simulink library "UndergraduateResearch"  (Simulink 8.1)
settings: Solver=ode45  StartTime=0.0  StopTime=10.0  RelTol=1e-3
undefined symbols (not defined in the file or in its folder): datafiI, datafiQ, i, magnitude
libraries: commchan3 x40, UndergraduateResearch x35, dspxfrm3 x6, dspstat3 x4, dspmtrx3 x4, commseqgen2 x4, dspindex x2, simulink x2, dspbuff3 x1
(part 2 of 2)

== system UndergraduateResearch/Frame Based Signal Generator (Any Sampling Frequency)/Noise Addition/AWGN channel16 ==
  Signal : Inport
  AWGN Channel : commchan3/AWGN Channel  InputProcessing=Columns as channels (frame based)  seed=16  noiseMode="Signal to noise ratio  (SNR)"  EbNodB=10  EsNodB=10  SNRdB=-20  bitsPerSym=1  Ps=1  Tsym=1  variance=1
  Frame Conversion : FrameConversion  OutFrame=Sample-based
  SIgnal+Noise : Outport
  wires:
  Signal/1 -> AWGN Channel/1
  AWGN Channel/1 -> Frame Conversion/1
  Frame Conversion/1 -> SIgnal+Noise/1

== system UndergraduateResearch/Frame Based Signal Generator (Any Sampling Frequency)/Noise Addition/AWGN channel17 ==
  Signal : Inport
  AWGN Channel : commchan3/AWGN Channel  InputProcessing=Columns as channels (frame based)  seed=17  noiseMode="Signal to noise ratio  (SNR)"  EbNodB=10  EsNodB=10  SNRdB=-20  bitsPerSym=1  Ps=1  Tsym=1  variance=1
  Frame Conversion : FrameConversion  OutFrame=Sample-based
  SIgnal+Noise : Outport
  wires:
  Signal/1 -> AWGN Channel/1
  AWGN Channel/1 -> Frame Conversion/1
  Frame Conversion/1 -> SIgnal+Noise/1

== system UndergraduateResearch/Frame Based Signal Generator (Any Sampling Frequency)/Noise Addition/AWGN channel18 ==
  Signal : Inport
  AWGN Channel : commchan3/AWGN Channel  InputProcessing=Columns as channels (frame based)  seed=18  noiseMode="Signal to noise ratio  (SNR)"  EbNodB=10  EsNodB=10  SNRdB=-20  bitsPerSym=1  Ps=1  Tsym=1  variance=1
  Frame Conversion : FrameConversion  OutFrame=Sample-based
  SIgnal+Noise : Outport
  wires:
  Signal/1 -> AWGN Channel/1
  AWGN Channel/1 -> Frame Conversion/1
  Frame Conversion/1 -> SIgnal+Noise/1

== system UndergraduateResearch/Frame Based Signal Generator (Any Sampling Frequency)/Noise Addition/AWGN channel19 ==
  Signal : Inport
  AWGN Channel : commchan3/AWGN Channel  InputProcessing=Columns as channels (frame based)  seed=19  noiseMode="Signal to noise ratio  (SNR)"  EbNodB=10  EsNodB=10  SNRdB=-20  bitsPerSym=1  Ps=1  Tsym=1  variance=1
  Frame Conversion : FrameConversion  OutFrame=Sample-based
  SIgnal+Noise : Outport
  wires:
  Signal/1 -> AWGN Channel/1
  AWGN Channel/1 -> Frame Conversion/1
  Frame Conversion/1 -> SIgnal+Noise/1

== system UndergraduateResearch/Frame Based Signal Generator (Any Sampling Frequency)/Noise Addition/AWGN channel2 ==
  Signal : Inport
  AWGN Channel : commchan3/AWGN Channel  InputProcessing=Columns as channels (frame based)  seed=2  noiseMode="Signal to noise ratio  (SNR)"  EbNodB=10  EsNodB=10  SNRdB=-20  bitsPerSym=1  Ps=1  Tsym=1  variance=1
  Frame Conversion : FrameConversion  OutFrame=Sample-based
  SIgnal+Noise : Outport
  wires:
  Signal/1 -> AWGN Channel/1
  AWGN Channel/1 -> Frame Conversion/1
  Frame Conversion/1 -> SIgnal+Noise/1

== system UndergraduateResearch/Frame Based Signal Generator (Any Sampling Frequency)/Noise Addition/AWGN channel20 ==
  Signal : Inport
  AWGN Channel : commchan3/AWGN Channel  InputProcessing=Columns as channels (frame based)  seed=20  noiseMode="Signal to noise ratio  (SNR)"  EbNodB=10  EsNodB=10  SNRdB=-20  bitsPerSym=1  Ps=1  Tsym=1  variance=1
  Frame Conversion : FrameConversion  OutFrame=Sample-based
  SIgnal+Noise : Outport
  wires:
  Signal/1 -> AWGN Channel/1
  AWGN Channel/1 -> Frame Conversion/1
  Frame Conversion/1 -> SIgnal+Noise/1

== system UndergraduateResearch/Frame Based Signal Generator (Any Sampling Frequency)/Noise Addition/AWGN channel21 ==
  Signal : Inport
  AWGN Channel : commchan3/AWGN Channel  InputProcessing=Columns as channels (frame based)  seed=21  noiseMode="Signal to noise ratio  (SNR)"  EbNodB=10  EsNodB=10  SNRdB=-20  bitsPerSym=1  Ps=1  Tsym=1  variance=1
  Frame Conversion : FrameConversion  OutFrame=Sample-based
  SIgnal+Noise : Outport
  wires:
  Signal/1 -> AWGN Channel/1
  AWGN Channel/1 -> Frame Conversion/1
  Frame Conversion/1 -> SIgnal+Noise/1

== system UndergraduateResearch/Frame Based Signal Generator (Any Sampling Frequency)/Noise Addition/AWGN channel22 ==
  Signal : Inport
  AWGN Channel : commchan3/AWGN Channel  InputProcessing=Columns as channels (frame based)  seed=22  noiseMode="Signal to noise ratio  (SNR)"  EbNodB=10  EsNodB=10  SNRdB=-20  bitsPerSym=1  Ps=1  Tsym=1  variance=1
  Frame Conversion : FrameConversion  OutFrame=Sample-based
  SIgnal+Noise : Outport
  wires:
  Signal/1 -> AWGN Channel/1
  AWGN Channel/1 -> Frame Conversion/1
  Frame Conversion/1 -> SIgnal+Noise/1

== system UndergraduateResearch/Frame Based Signal Generator (Any Sampling Frequency)/Noise Addition/AWGN channel23 ==
  Signal : Inport
  AWGN Channel : commchan3/AWGN Channel  InputProcessing=Columns as channels (frame based)  seed=23  noiseMode="Signal to noise ratio  (SNR)"  EbNodB=10  EsNodB=10  SNRdB=-20  bitsPerSym=1  Ps=1  Tsym=1  variance=1
  Frame Conversion : FrameConversion  OutFrame=Sample-based
  SIgnal+Noise : Outport
  wires:
  Signal/1 -> AWGN Channel/1
  AWGN Channel/1 -> Frame Conversion/1
  Frame Conversion/1 -> SIgnal+Noise/1

== system UndergraduateResearch/Frame Based Signal Generator (Any Sampling Frequency)/Noise Addition/AWGN channel24 ==
  Signal : Inport
  AWGN Channel : commchan3/AWGN Channel  InputProcessing=Columns as channels (frame based)  seed=24  noiseMode="Signal to noise ratio  (SNR)"  EbNodB=10  EsNodB=10  SNRdB=-20  bitsPerSym=1  Ps=1  Tsym=1  variance=1
  Frame Conversion : FrameConversion  OutFrame=Sample-based
  SIgnal+Noise : Outport
  wires:
  Signal/1 -> AWGN Channel/1
  AWGN Channel/1 -> Frame Conversion/1
  Frame Conversion/1 -> SIgnal+Noise/1

== system UndergraduateResearch/Frame Based Signal Generator (Any Sampling Frequency)/Noise Addition/AWGN channel25 ==
  Signal : Inport
  AWGN Channel : commchan3/AWGN Channel  InputProcessing=Columns as channels (frame based)  seed=25  noiseMode="Signal to noise ratio  (SNR)"  EbNodB=10  EsNodB=10  SNRdB=-20  bitsPerSym=1  Ps=1  Tsym=1  variance=1
  Frame Conversion : FrameConversion  OutFrame=Sample-based
  SIgnal+Noise : Outport
  wires:
  Signal/1 -> AWGN Channel/1
  AWGN Channel/1 -> Frame Conversion/1
  Frame Conversion/1 -> SIgnal+Noise/1

== system UndergraduateResearch/Frame Based Signal Generator (Any Sampling Frequency)/Noise Addition/AWGN channel26 ==
  Signal : Inport
  AWGN Channel : commchan3/AWGN Channel  InputProcessing=Columns as channels (frame based)  seed=26  noiseMode="Signal to noise ratio  (SNR)"  EbNodB=10  EsNodB=10  SNRdB=-20  bitsPerSym=1  Ps=1  Tsym=1  variance=1
  Frame Conversion : FrameConversion  OutFrame=Sample-based
  SIgnal+Noise : Outport
  wires:
  Signal/1 -> AWGN Channel/1
  AWGN Channel/1 -> Frame Conversion/1
  Frame Conversion/1 -> SIgnal+Noise/1

== system UndergraduateResearch/Frame Based Signal Generator (Any Sampling Frequency)/Noise Addition/AWGN channel27 ==
  Signal : Inport
  AWGN Channel : commchan3/AWGN Channel  InputProcessing=Columns as channels (frame based)  seed=27  noiseMode="Signal to noise ratio  (SNR)"  EbNodB=10  EsNodB=10  SNRdB=-20  bitsPerSym=1  Ps=1  Tsym=1  variance=1
  Frame Conversion : FrameConversion  OutFrame=Sample-based
  SIgnal+Noise : Outport
  wires:
  Signal/1 -> AWGN Channel/1
  AWGN Channel/1 -> Frame Conversion/1
  Frame Conversion/1 -> SIgnal+Noise/1

== system UndergraduateResearch/Frame Based Signal Generator (Any Sampling Frequency)/Noise Addition/AWGN channel28 ==
  Signal : Inport
  AWGN Channel : commchan3/AWGN Channel  InputProcessing=Columns as channels (frame based)  seed=28  noiseMode="Signal to noise ratio  (SNR)"  EbNodB=10  EsNodB=10  SNRdB=-20  bitsPerSym=1  Ps=1  Tsym=1  variance=1
  Frame Conversion : FrameConversion  OutFrame=Sample-based
  SIgnal+Noise : Outport
  wires:
  Signal/1 -> AWGN Channel/1
  AWGN Channel/1 -> Frame Conversion/1
  Frame Conversion/1 -> SIgnal+Noise/1

== system UndergraduateResearch/Frame Based Signal Generator (Any Sampling Frequency)/Noise Addition/AWGN channel29 ==
  Signal : Inport
  AWGN Channel : commchan3/AWGN Channel  InputProcessing=Columns as channels (frame based)  seed=29  noiseMode="Signal to noise ratio  (SNR)"  EbNodB=10  EsNodB=10  SNRdB=-20  bitsPerSym=1  Ps=1  Tsym=1  variance=1
  Frame Conversion : FrameConversion  OutFrame=Sample-based
  SIgnal+Noise : Outport
  wires:
  Signal/1 -> AWGN Channel/1
  AWGN Channel/1 -> Frame Conversion/1
  Frame Conversion/1 -> SIgnal+Noise/1

== system UndergraduateResearch/Frame Based Signal Generator (Any Sampling Frequency)/Noise Addition/AWGN channel3 ==
  Signal : Inport
  AWGN Channel : commchan3/AWGN Channel  InputProcessing=Columns as channels (frame based)  seed=3  noiseMode="Signal to noise ratio  (SNR)"  EbNodB=10  EsNodB=10  SNRdB=-20  bitsPerSym=1  Ps=1  Tsym=1  variance=1
  Frame Conversion : FrameConversion  OutFrame=Sample-based
  SIgnal+Noise : Outport
  wires:
  Signal/1 -> AWGN Channel/1
  AWGN Channel/1 -> Frame Conversion/1
  Frame Conversion/1 -> SIgnal+Noise/1

== system UndergraduateResearch/Frame Based Signal Generator (Any Sampling Frequency)/Noise Addition/AWGN channel30 ==
  Signal : Inport
  AWGN Channel : commchan3/AWGN Channel  InputProcessing=Columns as channels (frame based)  seed=10  noiseMode="Signal to noise ratio  (SNR)"  EbNodB=10  EsNodB=10  SNRdB=-20  bitsPerSym=1  Ps=1  Tsym=1  variance=1
  Frame Conversion : FrameConversion  OutFrame=Sample-based
  SIgnal+Noise : Outport
  wires:
  Signal/1 -> AWGN Channel/1
  AWGN Channel/1 -> Frame Conversion/1
  Frame Conversion/1 -> SIgnal+Noise/1

== system UndergraduateResearch/Frame Based Signal Generator (Any Sampling Frequency)/Noise Addition/AWGN channel31 ==
  Signal : Inport
  AWGN Channel : commchan3/AWGN Channel  InputProcessing=Columns as channels (frame based)  seed=10  noiseMode="Signal to noise ratio  (SNR)"  EbNodB=10  EsNodB=10  SNRdB=-20  bitsPerSym=1  Ps=1  Tsym=1  variance=1
  Frame Conversion : FrameConversion  OutFrame=Sample-based
  SIgnal+Noise : Outport
  wires:
  Signal/1 -> AWGN Channel/1
  AWGN Channel/1 -> Frame Conversion/1
  Frame Conversion/1 -> SIgnal+Noise/1

== system UndergraduateResearch/Frame Based Signal Generator (Any Sampling Frequency)/Noise Addition/AWGN channel32 ==
  Signal : Inport
  AWGN Channel : commchan3/AWGN Channel  InputProcessing=Columns as channels (frame based)  seed=10  noiseMode="Signal to noise ratio  (SNR)"  EbNodB=10  EsNodB=10  SNRdB=-20  bitsPerSym=1  Ps=1  Tsym=1  variance=1
  Frame Conversion : FrameConversion  OutFrame=Sample-based
  SIgnal+Noise : Outport
  wires:
  Signal/1 -> AWGN Channel/1
  AWGN Channel/1 -> Frame Conversion/1
  Frame Conversion/1 -> SIgnal+Noise/1

== system UndergraduateResearch/Frame Based Signal Generator (Any Sampling Frequency)/Noise Addition/AWGN channel33 ==
  Signal : Inport
  AWGN Channel : commchan3/AWGN Channel  InputProcessing=Columns as channels (frame based)  seed=10  noiseMode="Signal to noise ratio  (SNR)"  EbNodB=10  EsNodB=10  SNRdB=-20  bitsPerSym=1  Ps=1  Tsym=1  variance=1
  Frame Conversion : FrameConversion  OutFrame=Sample-based
  SIgnal+Noise : Outport
  wires:
  Signal/1 -> AWGN Channel/1
  AWGN Channel/1 -> Frame Conversion/1
  Frame Conversion/1 -> SIgnal+Noise/1

== system UndergraduateResearch/Frame Based Signal Generator (Any Sampling Frequency)/Noise Addition/AWGN channel34 ==
  Signal : Inport
  AWGN Channel : commchan3/AWGN Channel  InputProcessing=Columns as channels (frame based)  seed=10  noiseMode="Signal to noise ratio  (SNR)"  EbNodB=10  EsNodB=10  SNRdB=-20  bitsPerSym=1  Ps=1  Tsym=1  variance=1
  Frame Conversion : FrameConversion  OutFrame=Sample-based
  SIgnal+Noise : Outport
  wires:
  Signal/1 -> AWGN Channel/1
  AWGN Channel/1 -> Frame Conversion/1
  Frame Conversion/1 -> SIgnal+Noise/1

== system UndergraduateResearch/Frame Based Signal Generator (Any Sampling Frequency)/Noise Addition/AWGN channel35 ==
  Signal : Inport
  AWGN Channel : commchan3/AWGN Channel  InputProcessing=Columns as channels (frame based)  seed=10  noiseMode="Signal to noise ratio  (SNR)"  EbNodB=10  EsNodB=10  SNRdB=-20  bitsPerSym=1  Ps=1  Tsym=1  variance=1
  Frame Conversion : FrameConversion  OutFrame=Sample-based
  SIgnal+Noise : Outport
  wires:
  Signal/1 -> AWGN Channel/1
  AWGN Channel/1 -> Frame Conversion/1
  Frame Conversion/1 -> SIgnal+Noise/1

== system UndergraduateResearch/Frame Based Signal Generator (Any Sampling Frequency)/Noise Addition/AWGN channel36 ==
  Signal : Inport
  AWGN Channel : commchan3/AWGN Channel  InputProcessing=Columns as channels (frame based)  seed=10  noiseMode="Signal to noise ratio  (SNR)"  EbNodB=10  EsNodB=10  SNRdB=-20  bitsPerSym=1  Ps=1  Tsym=1  variance=1
  Frame Conversion : FrameConversion  OutFrame=Sample-based
  SIgnal+Noise : Outport
  wires:
  Signal/1 -> AWGN Channel/1
  AWGN Channel/1 -> Frame Conversion/1
  Frame Conversion/1 -> SIgnal+Noise/1

== system UndergraduateResearch/Frame Based Signal Generator (Any Sampling Frequency)/Noise Addition/AWGN channel37 ==
  Signal : Inport
  AWGN Channel : commchan3/AWGN Channel  InputProcessing=Columns as channels (frame based)  seed=10  noiseMode="Signal to noise ratio  (SNR)"  EbNodB=10  EsNodB=10  SNRdB=-20  bitsPerSym=1  Ps=1  Tsym=1  variance=1
  Frame Conversion : FrameConversion  OutFrame=Sample-based
  SIgnal+Noise : Outport
  wires:
  Signal/1 -> AWGN Channel/1
  AWGN Channel/1 -> Frame Conversion/1
  Frame Conversion/1 -> SIgnal+Noise/1

== system UndergraduateResearch/Frame Based Signal Generator (Any Sampling Frequency)/Noise Addition/AWGN channel38 ==
  Signal : Inport
  AWGN Channel : commchan3/AWGN Channel  InputProcessing=Columns as channels (frame based)  seed=10  noiseMode="Signal to noise ratio  (SNR)"  EbNodB=10  EsNodB=10  SNRdB=-20  bitsPerSym=1  Ps=1  Tsym=1  variance=1
  Frame Conversion : FrameConversion  OutFrame=Sample-based
  SIgnal+Noise : Outport
  wires:
  Signal/1 -> AWGN Channel/1
  AWGN Channel/1 -> Frame Conversion/1
  Frame Conversion/1 -> SIgnal+Noise/1

== system UndergraduateResearch/Frame Based Signal Generator (Any Sampling Frequency)/Noise Addition/AWGN channel39 ==
  Signal : Inport
  AWGN Channel : commchan3/AWGN Channel  InputProcessing=Columns as channels (frame based)  seed=10  noiseMode="Signal to noise ratio  (SNR)"  EbNodB=10  EsNodB=10  SNRdB=-20  bitsPerSym=1  Ps=1  Tsym=1  variance=1
  Frame Conversion : FrameConversion  OutFrame=Sample-based
  SIgnal+Noise : Outport
  wires:
  Signal/1 -> AWGN Channel/1
  AWGN Channel/1 -> Frame Conversion/1
  Frame Conversion/1 -> SIgnal+Noise/1

== system UndergraduateResearch/Frame Based Signal Generator (Any Sampling Frequency)/Noise Addition/AWGN channel4 ==
  Signal : Inport
  AWGN Channel : commchan3/AWGN Channel  InputProcessing=Columns as channels (frame based)  seed=10  noiseMode="Signal to noise ratio  (SNR)"  EbNodB=10  EsNodB=10  SNRdB=-20  bitsPerSym=1  Ps=1  Tsym=1  variance=1
  Frame Conversion : FrameConversion  OutFrame=Sample-based
  SIgnal+Noise : Outport
  wires:
  Signal/1 -> AWGN Channel/1
  AWGN Channel/1 -> Frame Conversion/1
  Frame Conversion/1 -> SIgnal+Noise/1

== system UndergraduateResearch/Frame Based Signal Generator (Any Sampling Frequency)/Noise Addition/AWGN channel40 ==
  Signal : Inport
  AWGN Channel : commchan3/AWGN Channel  InputProcessing=Columns as channels (frame based)  seed=10  noiseMode="Signal to noise ratio  (SNR)"  EbNodB=10  EsNodB=10  SNRdB=-20  bitsPerSym=1  Ps=1  Tsym=1  variance=1
  Frame Conversion : FrameConversion  OutFrame=Sample-based
  SIgnal+Noise : Outport
  wires:
  Signal/1 -> AWGN Channel/1
  AWGN Channel/1 -> Frame Conversion/1
  Frame Conversion/1 -> SIgnal+Noise/1

== system UndergraduateResearch/Frame Based Signal Generator (Any Sampling Frequency)/Noise Addition/AWGN channel5 ==
  Signal : Inport
  AWGN Channel : commchan3/AWGN Channel  InputProcessing=Columns as channels (frame based)  seed=10  noiseMode="Signal to noise ratio  (SNR)"  EbNodB=10  EsNodB=10  SNRdB=-20  bitsPerSym=1  Ps=1  Tsym=1  variance=1
  Frame Conversion : FrameConversion  OutFrame=Sample-based
  SIgnal+Noise : Outport
  wires:
  Signal/1 -> AWGN Channel/1
  AWGN Channel/1 -> Frame Conversion/1
  Frame Conversion/1 -> SIgnal+Noise/1

== system UndergraduateResearch/Frame Based Signal Generator (Any Sampling Frequency)/Noise Addition/AWGN channel6 ==
  Signal : Inport
  AWGN Channel : commchan3/AWGN Channel  InputProcessing=Columns as channels (frame based)  seed=10  noiseMode="Signal to noise ratio  (SNR)"  EbNodB=10  EsNodB=10  SNRdB=-20  bitsPerSym=1  Ps=1  Tsym=1  variance=1
  Frame Conversion : FrameConversion  OutFrame=Sample-based
  SIgnal+Noise : Outport
  wires:
  Signal/1 -> AWGN Channel/1
  AWGN Channel/1 -> Frame Conversion/1
  Frame Conversion/1 -> SIgnal+Noise/1

== system UndergraduateResearch/Frame Based Signal Generator (Any Sampling Frequency)/Noise Addition/AWGN channel7 ==
  Signal : Inport
  AWGN Channel : commchan3/AWGN Channel  InputProcessing=Columns as channels (frame based)  seed=10  noiseMode="Signal to noise ratio  (SNR)"  EbNodB=10  EsNodB=10  SNRdB=-20  bitsPerSym=1  Ps=1  Tsym=1  variance=1
  Frame Conversion : FrameConversion  OutFrame=Sample-based
  SIgnal+Noise : Outport
  wires:
  Signal/1 -> AWGN Channel/1
  AWGN Channel/1 -> Frame Conversion/1
  Frame Conversion/1 -> SIgnal+Noise/1

== system UndergraduateResearch/Frame Based Signal Generator (Any Sampling Frequency)/Noise Addition/AWGN channel8 ==
  Signal : Inport
  AWGN Channel : commchan3/AWGN Channel  InputProcessing=Columns as channels (frame based)  seed=10  noiseMode="Signal to noise ratio  (SNR)"  EbNodB=10  EsNodB=10  SNRdB=-20  bitsPerSym=1  Ps=1  Tsym=1  variance=1
  Frame Conversion : FrameConversion  OutFrame=Sample-based
  SIgnal+Noise : Outport
  wires:
  Signal/1 -> AWGN Channel/1
  AWGN Channel/1 -> Frame Conversion/1
  Frame Conversion/1 -> SIgnal+Noise/1

== system UndergraduateResearch/Frame Based Signal Generator (Any Sampling Frequency)/Noise Addition/AWGN channel9 ==
  Signal : Inport
  AWGN Channel : commchan3/AWGN Channel  InputProcessing=Columns as channels (frame based)  seed=10  noiseMode="Signal to noise ratio  (SNR)"  EbNodB=10  EsNodB=10  SNRdB=-20  bitsPerSym=1  Ps=1  Tsym=1  variance=1
  Frame Conversion : FrameConversion  OutFrame=Sample-based
  SIgnal+Noise : Outport
  wires:
  Signal/1 -> AWGN Channel/1
  AWGN Channel/1 -> Frame Conversion/1
  Frame Conversion/1 -> SIgnal+Noise/1

== matlab function Frame Based Signal Generator (Any Sampling Frequency)/BasebandSignal/CIRCSHIFT ==
  data: Signal input double; shiftedSignal output double; Shift input double
function shiftedSignal = CircularShift(Signal,Shift)
%#eml

shiftedSignal = circshift(Signal,Shift);

== matlab function Frame Based Signal Generator (Any Sampling Frequency)/BasebandSignal/CIRCSHIFT1 ==
  data: Signal input double; shiftedSignal output double; Shift input double
function shiftedSignal = CircularShift(Signal,Shift)
%#eml

shiftedSignal = circshift(Signal,Shift);

== matlab function Frame Based Signal Generator (Any Sampling Frequency)/BasebandSignal/CIRCSHIFT2 ==
  data: Signal input double; shiftedSignal output double; Shift input double
function shiftedSignal = CircularShift(Signal,Shift)
%#eml

shiftedSignal = circshift(Signal,Shift);

== matlab function Frame Based Signal Generator (Any Sampling Frequency)/BasebandSignal/CIRCSHIFT3 ==
  data: Signal input double; shiftedSignal output double; Shift input double
function shiftedSignal = CircularShift(Signal,Shift)
%#eml

shiftedSignal = circshift(Signal,Shift);

== matlab function Frame Based Signal Generator (Any Sampling Frequency)/BasebandSignal/CIRCSHIFT4 ==
  data: Signal input double; shiftedSignal output double; Shift input double
function shiftedSignal = CircularShift(Signal,Shift)
%#eml

shiftedSignal = circshift(Signal,Shift);

== matlab function Frame Based Signal Generator (Any Sampling Frequency)/BasebandSignal/CIRCSHIFT5 ==
  data: Signal input double; shiftedSignal output double; Shift input double
function shiftedSignal = CircularShift(Signal,Shift)
%#eml

shiftedSignal = circshift(Signal,Shift);

== matlab function Frame Based Signal Generator (Any Sampling Frequency)/BasebandSignal/CIRCSHIFT6 ==
  data: Signal input double; shiftedSignal output double; Shift input double
function shiftedSignal = CircularShift(Signal,Shift)
%#eml

shiftedSignal = circshift(Signal,Shift);

== matlab function Frame Based Signal Generator (Any Sampling Frequency)/BasebandSignal/CIRCSHIFT7 ==
  data: Signal input double; shiftedSignal output double; Shift input double
function shiftedSignal = CircularShift(Signal,Shift)
%#eml

shiftedSignal = circshift(Signal,Shift);

== matlab function Frame Based Signal Generator (Any Sampling Frequency)/BasebandSignal/CIRCSHIFT8 ==
  data: Signal input double; shiftedSignal output double; Shift input double
function shiftedSignal = CircularShift(Signal,Shift)
%#eml

shiftedSignal = circshift(Signal,Shift);

== matlab function Frame Based Signal Generator (Any Sampling Frequency)/BasebandSignal/MULTIPATH ==
  data: Signal input double; shiftedSignal output double; Shift input double
function shiftedSignal = CircularShift(Signal,Shift)
%#eml

shiftedSignal = circshift(Signal,Shift);

== matlab function CA CODE UPSAMPLER/ Selector ==
  data: Value output double; Index input double; Signal input double
function Value = Select_Element(Index,Signal)
%#codegen

    Value = Signal(Index,:);

== matlab function  Selector ==
  data: Value output double; Index input double; Signal input double
function Value = Select_Element(Index,Signal)
%#codegen

    Value = Signal(Index,:);

== matlab function CIRCSHIFT ==
  data: Signal input double; shiftedSignal output double; Shift input double
function shiftedSignal = CircularShift(Signal,Shift)
%#eml

shiftedSignal = circshift(Signal,Shift);

== matlab function Baseline Parallel Code Search (Doppler correction included)/Baseline Code Phase Acquisition Module/CIRCSHIFT ==
  data: Signal input double; shiftedSignal output double; Shift input double
function shiftedSignal = CircularShift(Signal,Shift)
%#eml

shiftedSignal = circshift(Signal,Shift);

== matlab function Baseline Parallel Code Search (Doppler correction included)/I and Q Separation/MATLAB Function ==
  data: u input double; u1 output double
function u1 = fcn(u)
%#codegen
u1 = u>0;

== matlab function Baseline Parallel Code Search (Doppler correction included)/I and Q Separation/MATLAB Function1 ==
  data: u input double; u1 output double
function u1 = fcn(u)
%#codegen
u1 = u>0;

== matlab function Baseline Parallel Code Search (Doppler correction included)/I and Q Separation/MATLAB Function2 ==
  data: u input double; u1 output double
function u1 = fcn(u)
%#codegen
u1=u>0;
